simulink model "sl_subsys_while1"  (Simulink 6.0)
settings: Solver=FixedStepDiscrete  StartTime=0.0  StopTime=10.0  FixedStep=1  RelTol=1e-3
settings Model: CovMetricSettings=d  Creator=The MathWorks Inc.  LastModifiedBy=batserve  ExtModeAutoUpdateStatusClock=off
settings OptimizationCC: BlockReduction=off  BooleanDataType=off
settings DebuggingCC: CheckExecutionContextPreStartOutputMsg=on  CheckExecutionContextRuntimeOutputMsg=on  SolverPrmCheckMsg=none
settings HardwareCC: TargetUnknown=on

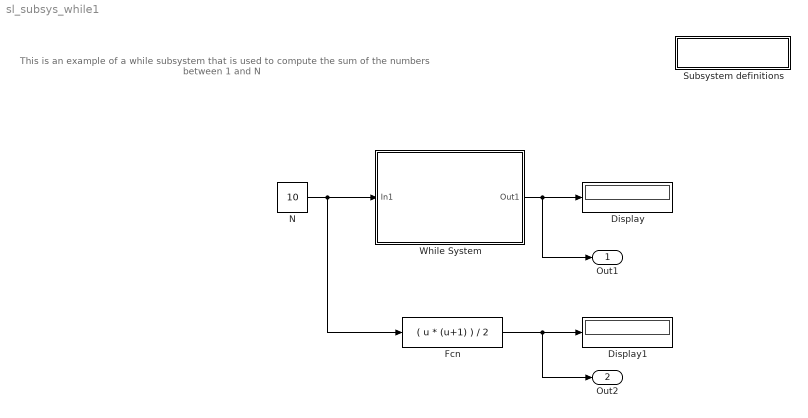
== system sl_subsys_while1 ==
  note: This is an example of a while subsystem that is used
      | to compute the sum of the numbers between 1 and N
  " Subsystem definitions" : Subsystem  PropExecContextAcrossSSBoundary=on
      settings: OpenFcn=helpview([matlabroot,'/toolbox/simulink/simdemos/sl_subsys_definitions.html']);
      mask Display: disp('Subsystem\ndefinitions')
  Display : Display
  Display1 : Display
  Fcn : Fcn  Expr=( u * (u+1) ) / 2
  N : Constant  Value=10
  While System : Subsystem  TreatAsAtomicUnit=on  PropExecContextAcrossSSBoundary=on
  Out1 : Outport
  Out2 : Outport  Port=2
  wires:
  N/1 -> While System/1(In1), Fcn/1
  While System/1(Out1) -> Display/1, Out1/1
  Fcn/1 -> Display1/1, Out2/1

== system sl_subsys_while1/ Subsystem definitions ==

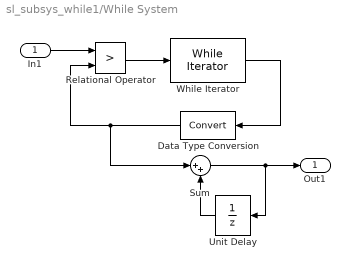
== system sl_subsys_while1/While System ==
  In1 : Inport  Port=1  LatchInput=off
  Data Type Conversion : DataTypeConversion  Orientation=left  OutDataTypeMode=double  SaturateOnIntegerOverflow=on  RndMeth=Zero
  Relational Operator : RelationalOperator  Operator=>  InputSameDT=on
  Sum : Sum  Inputs=|++  SaturateOnIntegerOverflow=on  InputSameDT=on
  Unit Delay : UnitDelay  Orientation=left  SampleTime=-1
  While Iterator : WhileIterator  MaxIters=-1  WhileBlockType=do-while  ResetStates=reset  ShowIterationPort=on
  Out1 : Outport
  wires:
  Sum/1 -> Unit Delay/1, Out1/1
  Relational Operator/1 -> While Iterator/1
  While Iterator/1 -> Data Type Conversion/1
  In1/1 -> Relational Operator/1
  Unit Delay/1 -> Sum/2
  Data Type Conversion/1 -> Relational Operator/2, Sum/1
